simulink model "CryoDet12Chan"  (R2016b)
settings: Solver=ode45  StartTime=0.0  StopTime=10e-4  MaxStep=1e-9  RelTol=1e-3
values from neighbouring files (symbols this model uses):
  Fclk = Fadc/2    (= 153600000)    [setupCryoFPGA.m]    (also in setupCryoNew.m)
  freqBusAddrBits = 4    [setupCryoFPGA.m]    (also in setupCryoNew.m)
  noise = exp(2i*pi*rand(1, noiseLen))    [setupCryoFPGA.m]    (also in setupCryoNew.m)
  noiseLen = 128    [setupCryoFPGA.m]    (also in setupCryoNew.m)
  noiseSteps = 32    [setupCryoFPGA.m]    (also in setupCryoNew.m)
  notch = tf( [1 a*wNotch/Q wNotch^2], [1 wNotch/Q wNotch^2])    [setupCryoFPGA.m]    (also in setupCryoNew.m)
  notch2 = tf( [1 a*wNotch/Q wNotch^2], [1 wNotch/Q wNotch^2])    [setupCryoFPGA.m]    (also in setupCryoNew.m)
  notch3 = tf( [1 a*wNotch/Q wNotch^2], [1 wNotch/Q wNotch^2])    [setupCryoFPGA.m]    (also in setupCryoNew.m)
  notch4 = tf( [1 a*wNotch/Q wNotch^2], [1 wNotch/Q wNotch^2])    [setupCryoFPGA.m]    (also in setupCryoNew.m)
  Tclk = 1/Fclk    (= 6.51041666667e-09)    [setupCryoFPGA.m]    (also in setupCryoNew.m)
undefined symbols (not defined in the file or in its folder): AXI4, Lite, xlipgetpartsetting
libraries: xbsIndex_r4 x1191
(part 4 of 9)

== system CryoDet12Chan/DspCore/AdcDac 0/eta/Complex Divide ==
  note: Complex multiplier has latency 6
  a_tvalid : Inport
  A_Q : Inport  Port=2
  A_I : Inport  Port=3
  b_tvalid : Inport  Port=4
  B_Q : Inport  Port=5
  B_I : Inport  Port=6
  AddSub : xbsIndex_r4/AddSub  mode=Addition  use_carryin=off  use_carryout=off  en=off  latency=3  precision=Full  arith_type="Signed  (2's comp)"  n_bits=48  bin_pt=44  quantization=Truncate  overflow=Flag as error  use_behavioral_HDL=on  hw_selection=Fabric  pipelined=off  dbl_ovrd=off  block_type=addsub
  CMult : xbsIndex_r4/CMult  const=-1  gui_display_data_type=Floating-point  const_n_bits=16  const_bin_pt=15  float_type=Single  exp_bits=8  fraction_bits=24  en=off  latency=3  precision=Full  arith_type="Signed  (2's comp)"  n_bits=32  bin_pt=30  quantization=Truncate  overflow=Wrap  use_behavioral_HDL=off  mem_type=Distributed RAM  pipeline=off  dbl_ovrd=off  block_type=cmult
  Constant : xbsIndex_r4/Constant  const=0  gui_display_data_type=Floating-point  arith_type=Floating-point  n_bits=63  bin_pt=15  preci_type=Single  exp_width=8  frac_width=24  explicit_period=off  period=1  equ=P=C  opselect=C  inp2=PCIN>>17  opr=+  inp1=P  carry=CIN  dbl_ovrd=off  block_type=constant
  Cplx Div 2 : Scope  NumInputPorts=3
  CplxProd : Subsystem
  Cpx Div : Scope  NumInputPorts=4
  Delay{,1..2,5} (4 alike) : xbsIndex_r4/Delay  rst=off  infoeditControl=Selection of Reset will increase slice count due to use of real FFs and instead of SRLs  en=off  latency=3  reg_retiming=on  dbl_ovrd=off  block_type=delay
  Delay3 : xbsIndex_r4/Delay  rst=off  infoeditControl=Selection of Reset will increase slice count due to use of real FFs and instead of SRLs  en=off  latency=8  reg_retiming=on  dbl_ovrd=off  block_type=delay
  Divide : xbsIndex_r4/Divide  flow_control=NonBlocking  axi_optimize_goal=Resources  algorithm_type=Radix2  infoedit1=Specify output fraction-width for Fixed-point division.  fractional_width=24  infoedit2=Specify latency for Floating-point division.  latency=8  rate=1  has_a_tlast=off  has_a_tuser=off  has_b_tlast=off  has_b_tuser=off  en=off  has_result_tready=off  result_tlast_behv=Pass_A_TLAST  has_underflow=on  has_overflow=on  has_invalid_op=on  has_divide_by_zero=on  fpo_op_type=mergeddivide  block_type=divide
      settings: infoedit=Blocking: Wait for data on all inputs, allow back-pressure.<br>NonBlocking: operate every cycle in which all inputs are valid, no back-pressure.
  Divide1 : xbsIndex_r4/Divide  flow_control=NonBlocking  axi_optimize_goal=Resources  algorithm_type=Radix2  infoedit1=Specify output fraction-width for Fixed-point division.  fractional_width=24  infoedit2=Specify latency for Floating-point division.  latency=8  rate=1  has_a_tlast=off  has_a_tuser=off  has_b_tlast=off  has_b_tuser=off  en=off  has_result_tready=off  result_tlast_behv=Pass_A_TLAST  has_underflow=on  has_overflow=on  has_invalid_op=on  has_divide_by_zero=on  fpo_op_type=mergeddivide  block_type=divide
      settings: infoedit=Blocking: Wait for data on all inputs, allow back-pressure.<br>NonBlocking: operate every cycle in which all inputs are valid, no back-pressure.
  Gateway Out{6..17} (12 alike) : xbsIndex_r4/Gateway Out  inherit_from_input=off  hdl_port=off  rows=1  columns=1  UseAsDAC=off  DACChannel='1'  interface=None  automatic_assignment=on  address_offset=hex2dec('00')  intf_name=''  intf_description=''  timing_constraint=None  locs_specified=off  LOCs={}  io_standard={}  block_type=gatewayout
  Mult : xbsIndex_r4/Mult  precision=Full  arith_type="Signed  (2's comp)"  n_bits=48  bin_pt=44  quantization=Truncate  overflow=Flag as error  en=off  latency=6  use_behavioral_HDL=on  opt=Speed  use_embedded=on  optimum_pipeline=on  pipeline=on  dbl_ovrd=off  use_rpm=on  placement_style=Triangular  block_type=mult
  Mult1 : xbsIndex_r4/Mult  precision=Full  arith_type="Signed  (2's comp)"  n_bits=48  bin_pt=44  quantization=Truncate  overflow=Flag as error  en=off  latency=6  use_behavioral_HDL=on  opt=Speed  use_embedded=on  optimum_pipeline=off  pipeline=on  dbl_ovrd=off  use_rpm=on  placement_style=Triangular  block_type=mult
  Mux{1,3..5,8..10} (7 alike) : Mux  Inputs=2
  Mux6 : xbsIndex_r4/Mux  inputs=2  en=off  latency=0  precision=Full  arith_type=Unsigned  n_bits=63  bin_pt=15  quantization=Truncate  overflow=Flag as error  dbl_ovrd=off  block_type=mux
  Mux7 : xbsIndex_r4/Mux  inputs=2  en=off  latency=0  precision=Full  arith_type=Unsigned  n_bits=63  bin_pt=15  quantization=Truncate  overflow=Flag as error  dbl_ovrd=off  block_type=mux
  Terminator5 : Terminator
  tvalidOut : Outport
  Out_Q : Outport  Port=2
  Out_I : Outport  Port=3
  invalid op : Outport  Port=4
  wires:
  a_tvalid/1 -> Gateway Out13/1, Gateway Out12/1, Delay/1
  A_Q/1 -> Delay1/1, Gateway Out14/1
  A_I/1 -> Delay2/1, Gateway Out15/1
  Divide/1 -> Mux7/2
  Mult1/1 -> AddSub/2
  AddSub/1 -> Divide/2, Divide1/2
  Divide1/4 -> Gateway Out11/1, invalid op/1, Mux6/1, Mux7/1
  Mux7/1 -> Gateway Out6/1, Out_Q/1
  Mux6/1 -> Out_I/1, Gateway Out7/1
  Mult/1 -> AddSub/1
  Gateway Out6/1 -> Mux3/1
  Gateway Out7/1 -> Mux3/2
  Gateway Out8/1 -> Mux4/1
  Gateway Out9/1 -> Mux4/2
  Gateway Out10/1 -> Mux5/1
  Gateway Out11/1 -> Mux5/2
  Divide1/1 -> Mux6/2
  Constant/1 -> Mux7/3, Mux6/3
  Delay5/1 -> CplxProd/5(Re_B)
  Delay2/1 -> CplxProd/3(Re_A)
  Delay1/1 -> CplxProd/2(Im_A)
  Delay/1 -> CplxProd/1(tvalidIn)
  B_Q/1 -> Mult1/1, Mult1/2, Gateway Out16/1, CMult/1
  B_I/1 -> Mult/1, Mult/2, Delay5/1, Gateway Out17/1
  CMult/1 -> CplxProd/4(Im_B)
  Gateway Out12/1 -> Mux8/1
  Gateway Out13/1 -> Mux8/2
  Gateway Out14/1 -> Mux9/1
  Gateway Out15/1 -> Mux9/2
  Gateway Out16/1 -> Mux10/1
  Gateway Out17/1 -> Mux10/2
  Mux8/1 -> Cplx Div 2/1
  Mux9/1 -> Cplx Div 2/2
  Mux10/1 -> Cplx Div 2/3
  b_tvalid/1 -> Terminator5/1
  CplxProd/2(Im_Out) -> Divide/1
  CplxProd/1(tvalidOut) -> Mux1/2, Delay3/1
  CplxProd/3(Re_Out) -> Divide1/1
  Divide1/2 -> Gateway Out8/1
  Divide1/3 -> Gateway Out9/1
  Divide1/5 -> Gateway Out10/1
  Mux3/1 -> Cpx Div/2
  Mux4/1 -> Cpx Div/3
  Mux5/1 -> Cpx Div/4
  Delay3/1 -> Mux1/1, tvalidOut/1
  Mux1/1 -> Cpx Div/1

== system CryoDet12Chan/DspCore/AdcDac 0/eta/CplxProd ==
  tvalidIn : Inport
  Im_A : Inport  Port=2
  Re_A : Inport  Port=3
  Im_B : Inport  Port=4
  Re_B : Inport  Port=5
  AddSub : xbsIndex_r4/AddSub  mode=Subtraction  use_carryin=off  use_carryout=off  en=off  latency=3  precision=Full  arith_type=Unsigned  n_bits=16  bin_pt=14  quantization=Truncate  overflow=Wrap  use_behavioral_HDL=off  hw_selection=DSP48  pipelined=on  dbl_ovrd=off  block_type=addsub
  AddSub1 : xbsIndex_r4/AddSub  mode=Addition  use_carryin=off  use_carryout=off  en=off  latency=3  precision=Full  arith_type=Unsigned  n_bits=16  bin_pt=14  quantization=Truncate  overflow=Wrap  use_behavioral_HDL=off  hw_selection=DSP48  pipelined=on  dbl_ovrd=off  block_type=addsub
  Delay : xbsIndex_r4/Delay  rst=off  infoeditControl=Selection of Reset will increase slice count due to use of real FFs and instead of SRLs  en=off  latency=3  reg_retiming=off  dbl_ovrd=off  block_type=delay
  Delay1 : xbsIndex_r4/Delay  rst=off  infoeditControl=Selection of Reset will increase slice count due to use of real FFs and instead of SRLs  en=off  latency=3  reg_retiming=off  dbl_ovrd=off  block_type=delay
  Mult{,1..3} (4 alike) : xbsIndex_r4/Mult  precision=Full  arith_type="Signed  (2's comp)"  n_bits=16  bin_pt=14  quantization=Truncate  overflow=Wrap  en=off  latency=3  use_behavioral_HDL=off  opt=Speed  use_embedded=on  optimum_pipeline=off  pipeline=on  dbl_ovrd=off  use_rpm=on  placement_style=Triangular  block_type=mult
  tvalidOut : Outport
  Im_Out : Outport  Port=2
  Re_Out : Outport  Port=3
  wires:
  Delay/1 -> Delay1/1
  Mult2/1 -> AddSub1/1
  Mult/1 -> AddSub/1
  Mult1/1 -> AddSub/2
  Mult3/1 -> AddSub1/2
  Re_A/1 -> Mult3/1, Mult/1
  Im_A/1 -> Mult2/1, Mult1/1
  tvalidIn/1 -> Delay/1
  Im_B/1 -> Mult1/2, Mult3/2
  Re_B/1 -> Mult/2, Mult2/2
  Delay1/1 -> tvalidOut/1
  AddSub/1 -> Re_Out/1
  AddSub1/1 -> Im_Out/1

== system CryoDet12Chan/DspCore/AdcDac 0/eta/CplxProd1 ==
  tvalidIn : Inport
  Im_A : Inport  Port=2
  Re_A : Inport  Port=3
  Im_B : Inport  Port=4
  Re_B : Inport  Port=5
  AddSub : xbsIndex_r4/AddSub  mode=Subtraction  use_carryin=off  use_carryout=off  en=off  latency=3  precision=Full  arith_type=Unsigned  n_bits=16  bin_pt=14  quantization=Truncate  overflow=Wrap  use_behavioral_HDL=off  hw_selection=DSP48  pipelined=on  dbl_ovrd=off  block_type=addsub
  AddSub1 : xbsIndex_r4/AddSub  mode=Addition  use_carryin=off  use_carryout=off  en=off  latency=3  precision=Full  arith_type=Unsigned  n_bits=16  bin_pt=14  quantization=Truncate  overflow=Wrap  use_behavioral_HDL=off  hw_selection=DSP48  pipelined=on  dbl_ovrd=off  block_type=addsub
  Delay : xbsIndex_r4/Delay  rst=off  infoeditControl=Selection of Reset will increase slice count due to use of real FFs and instead of SRLs  en=off  latency=3  reg_retiming=off  dbl_ovrd=off  block_type=delay
  Delay1 : xbsIndex_r4/Delay  rst=off  infoeditControl=Selection of Reset will increase slice count due to use of real FFs and instead of SRLs  en=off  latency=3  reg_retiming=off  dbl_ovrd=off  block_type=delay
  Mult{,1..3} (4 alike) : xbsIndex_r4/Mult  precision=Full  arith_type="Signed  (2's comp)"  n_bits=16  bin_pt=14  quantization=Truncate  overflow=Wrap  en=off  latency=3  use_behavioral_HDL=off  opt=Speed  use_embedded=on  optimum_pipeline=off  pipeline=on  dbl_ovrd=off  use_rpm=on  placement_style=Triangular  block_type=mult
  tvalidOut : Outport
  Im_Out : Outport  Port=2
  Re_Out : Outport  Port=3
  wires:
  Delay/1 -> Delay1/1
  Mult2/1 -> AddSub1/1
  Mult/1 -> AddSub/1
  Mult1/1 -> AddSub/2
  Mult3/1 -> AddSub1/2
  Re_A/1 -> Mult3/1, Mult/1
  Im_A/1 -> Mult2/1, Mult1/1
  tvalidIn/1 -> Delay/1
  Im_B/1 -> Mult1/2, Mult3/2
  Re_B/1 -> Mult/2, Mult2/2
  Delay1/1 -> tvalidOut/1
  AddSub/1 -> Re_Out/1
  AddSub1/1 -> Im_Out/1

== system CryoDet12Chan/DspCore/AdcDac 0/eta/CplxProd2 ==
  tvalidIn : Inport
  Im_A : Inport  Port=2
  Re_A : Inport  Port=3
  Im_B : Inport  Port=4
  Re_B : Inport  Port=5
  AddSub : xbsIndex_r4/AddSub  mode=Subtraction  use_carryin=off  use_carryout=off  en=off  latency=3  precision=Full  arith_type=Unsigned  n_bits=16  bin_pt=14  quantization=Truncate  overflow=Wrap  use_behavioral_HDL=off  hw_selection=DSP48  pipelined=on  dbl_ovrd=off  block_type=addsub
  AddSub1 : xbsIndex_r4/AddSub  mode=Addition  use_carryin=off  use_carryout=off  en=off  latency=3  precision=Full  arith_type=Unsigned  n_bits=16  bin_pt=14  quantization=Truncate  overflow=Wrap  use_behavioral_HDL=off  hw_selection=DSP48  pipelined=on  dbl_ovrd=off  block_type=addsub
  Delay : xbsIndex_r4/Delay  rst=off  infoeditControl=Selection of Reset will increase slice count due to use of real FFs and instead of SRLs  en=off  latency=3  reg_retiming=off  dbl_ovrd=off  block_type=delay
  Delay1 : xbsIndex_r4/Delay  rst=off  infoeditControl=Selection of Reset will increase slice count due to use of real FFs and instead of SRLs  en=off  latency=3  reg_retiming=off  dbl_ovrd=off  block_type=delay
  Mult{,1..3} (4 alike) : xbsIndex_r4/Mult  precision=Full  arith_type="Signed  (2's comp)"  n_bits=16  bin_pt=14  quantization=Truncate  overflow=Wrap  en=off  latency=3  use_behavioral_HDL=off  opt=Speed  use_embedded=on  optimum_pipeline=off  pipeline=on  dbl_ovrd=off  use_rpm=on  placement_style=Triangular  block_type=mult
  tvalidOut : Outport
  Im_Out : Outport  Port=2
  Re_Out : Outport  Port=3
  wires:
  Delay/1 -> Delay1/1
  Mult2/1 -> AddSub1/1
  Mult/1 -> AddSub/1
  Mult1/1 -> AddSub/2
  Mult3/1 -> AddSub1/2
  Re_A/1 -> Mult3/1, Mult/1
  Im_A/1 -> Mult2/1, Mult1/1
  tvalidIn/1 -> Delay/1
  Im_B/1 -> Mult1/2, Mult3/2
  Re_B/1 -> Mult/2, Mult2/2
  Delay1/1 -> tvalidOut/1
  AddSub/1 -> Re_Out/1
  AddSub1/1 -> Im_Out/1

== system CryoDet12Chan/DspCore/AdcDac 0/eta/LPF ==
  note: REF channel should not be low-passed!
      | Needs to have same bandwidth as signal channel
      | but latency must match
  note: streaming interface? so complex divide gets data at lower rate?
  note: tvalid
  note: Channel #
  note: Sig+
  note: Sig-
  note: Ref+
  note: Ref
  note: Sig
  note: Ref-
  In1 : Inport
  Bus Creator : BusCreator  Inputs=2
  Bus Creator1 : BusCreator  Inputs=2
  Bus Selector : BusSelector  OutputSignals=chanAndTvalid,signal2
  Bus Selector1 : BusSelector  OutputSignals=channel,valid
  Bus Selector2 : BusSelector  OutputSignals=channel,tvalid
  CIC Compiler 4.0 {1..10} (10 alike) : xbsIndex_r4/CIC Compiler 4.0   filter_type=Decimation  number_of_stages=3  differential_delay=1  number_of_channels=12  sample_rate_changes=Fixed  fixed_or_initial_rate=8  minimum_rate=8  maximum_rate=8  ratespecification=Sample_Period  sampleperiod=1  hardwareoversamplingrate=1  quantization=Truncation  output_data_width=24  use_xtreme_dsp_slice=off  use_streaming_interface=on  has_aclken=off  has_aresetn=on  has_dout_tready=off  trim_axipin_name=on  gui_behaviour=Sysgen_GUI  input_data_width=18  ip_name=CIC Compiler  ip_version=4.0  dsptool_ready=true  wrapper_available=true  port_translation_map={ 'aclken' => 'en', 'aresetn' => 'rst' }  ipcore_xco_need_fpga_part=true  ipcore_verbose=false  block_type=cic_compiler_v4_0
  CIC LPF Scope : Scope  NumInputPorts=6
  CIC LPF input scope : Scope  NumInputPorts=5
  CIC reset : Subsystem
  Constant4 : xbsIndex_r4/Constant  const=10  gui_display_data_type=Fixed-point  arith_type=Unsigned  n_bits=4  bin_pt=0  preci_type=Single  exp_width=8  frac_width=24  explicit_period=off  period=1  equ=P=C  opselect=C  inp2=PCIN>>17  opr=+  inp1=P  carry=CIN  dbl_ovrd=off  block_type=constant
  Demux{,3..6} (5 alike) : Demux  Outputs=2
  Demux1 : Demux  Outputs=6
  Display : Display
  Gateway Out{,1,5..18} (16 alike) : xbsIndex_r4/Gateway Out  inherit_from_input=off  hdl_port=off  rows=1  columns=1  UseAsDAC=off  DACChannel='1'  interface=None  automatic_assignment=on  address_offset=hex2dec('00')  intf_name=''  intf_description=''  timing_constraint=None  locs_specified=off  LOCs={}  io_standard={}  block_type=gatewayout
  LPF chan output : Scope  NumInputPorts=2
  Mux : Mux  Inputs=2
  Mux1 : Mux  Inputs=10
  Mux3 : Mux  Inputs=2
  Mux4 : Mux  Inputs=2
  Scale{,1..9} (10 alike) : xbsIndex_r4/Scale  scale_factor=-9  dbl_ovrd=off  block_type=scale
  Terminator : Terminator
  Out1 : Outport
  wires:
  Demux1/1 -> Terminator/1
  Demux1/2 -> Demux/1
  Demux1/3 -> Demux3/1
  Demux1/5 -> Demux5/1
  Demux1/6 -> Demux6/1
  Bus Selector/2 -> Demux1/1  "<signal2>"
  In1/1 -> Bus Selector/1
  Demux1/4 -> Demux4/1
  Demux/1 -> Gateway Out16/1, CIC Compiler 4.0 3/2
  Demux/2 -> CIC Compiler 4.0 1/2
  Demux3/1 -> CIC Compiler 4.0 2/2
  Demux3/2 -> CIC Compiler 4.0 4/2
  Demux5/1 -> CIC Compiler 4.0 7/2
  Demux5/2 -> CIC Compiler 4.0 8/2
  Demux6/1 -> CIC Compiler 4.0 9/2
  Demux6/2 -> CIC Compiler 4.0 10/2
  Bus Selector1/2 -> CIC Compiler 4.0 3/1, CIC Compiler 4.0 1/1, CIC Compiler 4.0 2/1, CIC Compiler 4.0 4/1, CIC Compiler 4.0 5/1, CIC Compiler 4.0 6/1, CIC Compiler 4.0 7/1, CIC Compiler 4.0 8/1, CIC Compiler 4.0 9/1, CIC Compiler 4.0 10/1  "<valid>"
  Bus Selector1/1 -> Gateway Out15/1, CIC reset/2(Channel), [ChanIn]  "<channel>"
  Bus Selector/1 -> Bus Selector1/1  "<chanAndTvalid>"
  CIC Compiler 4.0 3/3 -> Scale/1
  CIC Compiler 4.0 1/3 -> Scale1/1
  CIC Compiler 4.0 2/3 -> Scale2/1
  CIC Compiler 4.0 4/3 -> Scale3/1
  Demux4/1 -> CIC Compiler 4.0 5/2
  Demux4/2 -> CIC Compiler 4.0 6/2
  CIC Compiler 4.0 7/3 -> Scale4/1
  CIC Compiler 4.0 8/3 -> Scale5/1
  CIC Compiler 4.0 9/3 -> Scale6/1
  CIC Compiler 4.0 10/3 -> Scale7/1
  Mux1/1 -> Bus Creator/2
  Bus Creator/1 -> Out1/1
  Bus Creator1/1 -> Bus Creator/1, Bus Selector2/1
  Scale/1 -> Gateway Out1/1, Mux1/1
  Scale1/1 -> Mux1/2
  Scale2/1 -> Mux1/3
  Scale3/1 -> Mux1/4
  Scale4/1 -> Mux1/7
  Scale5/1 -> Mux1/8
  Scale6/1 -> Mux1/9
  Scale7/1 -> Mux1/10
  CIC Compiler 4.0 7/2 -> Bus Creator1/2  "tvalid"
  Scale8/1 -> Mux1/5
  Scale9/1 -> Mux1/6
  CIC Compiler 4.0 4/6 -> Gateway Out/1
  CIC Compiler 4.0 7/6 -> Bus Creator1/1  "channel"
  CIC Compiler 4.0 3/1 -> Gateway Out5/1
  CIC Compiler 4.0 3/2 -> Gateway Out6/1
  CIC Compiler 4.0 3/4 -> Gateway Out7/1
  CIC Compiler 4.0 3/5 -> Gateway Out8/1
  CIC Compiler 4.0 3/6 -> Gateway Out9/1
  CIC Compiler 4.0 3/7 -> Gateway Out10/1
  CIC Compiler 4.0 3/8 -> Gateway Out11/1
  Gateway Out11/1 -> Mux3/2
  Gateway Out10/1 -> Mux3/1
  Mux3/1 -> CIC LPF Scope/6
  Gateway Out9/1 -> CIC LPF Scope/5
  Gateway Out8/1 -> CIC LPF Scope/4
  Gateway Out7/1 -> CIC LPF Scope/3
  Gateway Out6/1 -> CIC LPF Scope/2
  CIC reset/1(notResetOut) -> Gateway Out18/1, CIC Compiler 4.0 3/4, CIC Compiler 4.0 1/4, CIC Compiler 4.0 2/4, CIC Compiler 4.0 4/4, CIC Compiler 4.0 5/4, CIC Compiler 4.0 6/4, CIC Compiler 4.0 7/4, CIC Compiler 4.0 8/4, CIC Compiler 4.0 9/4, CIC Compiler 4.0 10/4
  Constant4/1 -> CIC reset/3(N-2)
  [fpgaReset] -> Gateway Out14/1, CIC reset/1(resetIn)
  CIC reset/2(tlast) -> CIC Compiler 4.0 2/3, CIC Compiler 4.0 5/3, CIC Compiler 4.0 6/3, CIC Compiler 4.0 8/3, CIC Compiler 4.0 9/3, CIC Compiler 4.0 10/3, CIC Compiler 4.0 7/3, CIC Compiler 4.0 4/3, CIC Compiler 4.0 3/3, Gateway Out17/1, CIC Compiler 4.0 1/3
  Gateway Out18/1 -> CIC LPF input scope/5
  Gateway Out17/1 -> CIC LPF input scope/4
  Gateway Out16/1 -> CIC LPF input scope/3
  Gateway Out15/1 -> CIC LPF input scope/2
  Gateway Out14/1 -> CIC LPF input scope/1
  Gateway Out5/1 -> Mux4/2
  Gateway Out1/1 -> Mux4/1
  Mux4/1 -> CIC LPF Scope/1
  Bus Selector2/2 -> Gateway Out13/1  "<tvalid>"
  Bus Selector2/1 -> Gateway Out12/1  "<channel>"
  Gateway Out12/1 -> Mux/1
  Gateway Out13/1 -> Mux/2
  Mux/1 -> LPF chan output/1
  Gateway Out/1 -> LPF chan output/2, Display/1
  CIC Compiler 4.0 5/3 -> Scale8/1
  CIC Compiler 4.0 6/3 -> Scale9/1

== system CryoDet12Chan/DspCore/AdcDac 0/loopFilter/initial Frequencies ==
  note: Channel 15 used for none of above
  note: initial Frequencies
  note: select initial frequency
      | for now just mux from input registers
      | eventually configure RAM and loading protocol
  channel : Inport
  Gateway Out12 : xbsIndex_r4/Gateway Out  inherit_from_input=off  hdl_port=off  rows=1  columns=1  UseAsDAC=off  DACChannel='1'  interface=None  automatic_assignment=on  address_offset=hex2dec('00')  intf_name=''  intf_description=''  timing_constraint=None  locs_specified=off  LOCs={}  io_standard={}  block_type=gatewayout
  Gateway Out13 : xbsIndex_r4/Gateway Out  inherit_from_input=off  hdl_port=off  rows=1  columns=1  UseAsDAC=off  DACChannel='1'  interface=None  automatic_assignment=on  address_offset=hex2dec('00')  intf_name=''  intf_description=''  timing_constraint=None  locs_specified=off  LOCs={}  io_standard={}  block_type=gatewayout
  Mux : xbsIndex_r4/Mux  inputs=16  en=off  latency=0  precision=Full  arith_type=Unsigned  n_bits=24  bin_pt=24  quantization=Truncate  overflow=Wrap  dbl_ovrd=off  block_type=mux
  initial Freqs : Scope  NumInputPorts=2
  Fi : Outport
  wires:
  channel/1 -> Gateway Out12/1, Mux/1
  [F0] -> Mux/2
  [F1] -> Mux/3
  [F2] -> Mux/4
  [F3] -> Mux/5
  [F4] -> Mux/6
  [F5] -> Mux/7
  [F6] -> Mux/8
  [F7] -> Mux/9
  [F8] -> Mux/10
  [F9] -> Mux/11
  [F10] -> Mux/12
  [F11] -> Mux/14, Mux/15, Mux/16, Mux/17, Mux/13
  Mux/1 -> Gateway Out13/1, Fi/1
  Gateway Out13/1 -> initial Freqs/2
  Gateway Out12/1 -> initial Freqs/1

== system CryoDet12Chan/DspCore/AdcDac 0/twelveLineUDC 0/DAC Sum ==
  note: Final adder stages reduce to 16 bits
  note: DAC1 (odd samples)
  note: DAC0 (even samples)
  In1 : Inport
  In2 : Inport  Port=2
  In3 : Inport  Port=3
  In4 : Inport  Port=4
  In5 : Inport  Port=5
  In6 : Inport  Port=6
  In7 : Inport  Port=7
  In8 : Inport  Port=8
  In9 : Inport  Port=9
  In10 : Inport  Port=10
  In11 : Inport  Port=11
  In12 : Inport  Port=12
  AddSub{,1..19} (20 alike) : xbsIndex_r4/AddSub  mode=Addition  use_carryin=off  use_carryout=off  en=off  latency=3  precision=User Defined  arith_type="Signed  (2's comp)"  n_bits=20  bin_pt=15  quantization=Truncate  overflow=Wrap  use_behavioral_HDL=off  hw_selection=Fabric  pipelined=off  dbl_ovrd=off  block_type=addsub
  AddSub20 : xbsIndex_r4/AddSub  mode=Addition  use_carryin=off  use_carryout=off  en=off  latency=3  precision=User Defined  arith_type="Signed  (2's comp)"  n_bits=16  bin_pt=15  quantization="Round  (unbiased: +/- Inf)"  overflow=Saturate  use_behavioral_HDL=off  hw_selection=Fabric  pipelined=off  dbl_ovrd=off  block_type=addsub
  AddSub21 : xbsIndex_r4/AddSub  mode=Addition  use_carryin=off  use_carryout=off  en=off  latency=3  precision=User Defined  arith_type="Signed  (2's comp)"  n_bits=16  bin_pt=15  quantization="Round  (unbiased: +/- Inf)"  overflow=Saturate  use_behavioral_HDL=off  hw_selection=Fabric  pipelined=off  dbl_ovrd=off  block_type=addsub
  DAC sum scope : Scope  NumInputPorts=2
  DAC sum scope1 : Scope  NumInputPorts=6
  Demux{,1..11} (12 alike) : Demux  Outputs=2
  Gateway Out{,1..9} (10 alike) : xbsIndex_r4/Gateway Out  inherit_from_input=off  hdl_port=off  rows=1  columns=1  UseAsDAC=off  DACChannel='1'  interface=None  automatic_assignment=on  address_offset=hex2dec('00')  intf_name=''  intf_description=''  timing_constraint=None  locs_specified=off  LOCs={}  io_standard={}  block_type=gatewayout
  Mux : Mux  Inputs=2
  Mux1 : Mux  Inputs=2
  Mux2 : Mux  Inputs=2
  Out1 : Outport
  wires:
  In1/1 -> Demux1/1
  In2/1 -> Demux/1
  In3/1 -> Demux2/1
  In4/1 -> Demux3/1
  In5/1 -> Demux4/1
  In6/1 -> Demux5/1
  In7/1 -> Demux6/1
  In8/1 -> Demux7/1
  In9/1 -> Demux8/1
  In10/1 -> Demux9/1
  In11/1 -> Demux10/1
  Demux/1 -> Gateway Out5/1, AddSub/2
  Demux2/1 -> Gateway Out6/1, AddSub2/1
  Demux3/1 -> Gateway Out7/1, AddSub2/2
  Demux4/1 -> Gateway Out8/1, AddSub4/1
  Demux5/1 -> Gateway Out9/1, AddSub4/2
  Demux6/1 -> AddSub6/1
  Demux8/1 -> AddSub8/1
  In12/1 -> Demux11/1
  AddSub20/1 -> Mux/1
  AddSub21/1 -> Mux/2
  Mux/1 -> Out1/1
  Demux7/1 -> AddSub6/2
  Demux9/1 -> AddSub8/2
  Demux10/1 -> AddSub10/1
  Demux11/1 -> AddSub10/2
  Demux/2 -> AddSub1/1
  Demux1/2 -> AddSub1/2
  Demux11/2 -> AddSub11/1
  Demux10/2 -> AddSub11/2
  Demux9/2 -> AddSub9/1
  Demux8/2 -> AddSub9/2
  Demux7/2 -> AddSub7/1
  Demux6/2 -> AddSub7/2
  Demux5/2 -> AddSub5/1
  Demux4/2 -> AddSub5/2
  Demux3/2 -> AddSub3/1
  Demux2/2 -> AddSub3/2
  AddSub/1 -> AddSub12/1
  AddSub2/1 -> AddSub12/2
  AddSub4/1 -> AddSub13/1
  AddSub6/1 -> AddSub13/2
  AddSub8/1 -> AddSub14/1
  AddSub10/1 -> AddSub14/2
  AddSub12/1 -> AddSub15/1
  AddSub13/1 -> AddSub15/2
  AddSub15/1 -> AddSub20/1, Gateway Out/1
  AddSub14/1 -> Gateway Out1/1, AddSub20/2
  AddSub1/1 -> AddSub16/1
  AddSub3/1 -> AddSub16/2
  AddSub5/1 -> AddSub17/1
  AddSub7/1 -> AddSub17/2
  AddSub9/1 -> AddSub18/1
  AddSub11/1 -> AddSub18/2
  AddSub16/1 -> AddSub19/1
  AddSub17/1 -> AddSub19/2
  AddSub19/1 -> Gateway Out2/1, AddSub21/1
  AddSub18/1 -> AddSub21/2, Gateway Out3/1
  Gateway Out3/1 -> Mux2/2
  Gateway Out2/1 -> Mux2/1
  Gateway Out1/1 -> Mux1/2
  Gateway Out/1 -> Mux1/1
  Mux1/1 -> DAC sum scope/1
  Mux2/1 -> DAC sum scope/2
  Gateway Out4/1 -> DAC sum scope1/1
  Gateway Out5/1 -> DAC sum scope1/2
  Gateway Out6/1 -> DAC sum scope1/3
  Gateway Out7/1 -> DAC sum scope1/4
  Gateway Out8/1 -> DAC sum scope1/5
  Gateway Out9/1 -> DAC sum scope1/6
  Demux1/1 -> Gateway Out4/1, AddSub/1

== system CryoDet12Chan/DspCore/AdcDac 0/twelveLineUDC 0/Mux12X4 ==
  note: I think this will select a channel 1 or 2 ticks after it has updated,
      | which should work fine. But optimal would be to delay synch in by 11 ticks = N-1
  note: Channel ID
  note: Reference Q&I
  note: Signal Q&I
  note: Twelve busses 4-wide each time-division multiplexed onto a 4-wide bus
  line0 : Inport
  line1 : Inport  Port=2
  line2 : Inport  Port=3
  line3 : Inport  Port=4
  line4 : Inport  Port=5
  line5 : Inport  Port=6
  line6 : Inport  Port=7
  line7 : Inport  Port=8
  line8 : Inport  Port=9
  line9 : Inport  Port=10
  line10 : Inport  Port=11
  line11 : Inport  Port=12
  synch : Inport  Port=13
  "12x4 Mux out scope " : Scope  NumInputPorts=3
  Bus Creator : BusCreator  Inputs=2
  Counter : xbsIndex_r4/Counter  cnt_type=Count Limited  cnt_to=11  operation=Up  start_count=0  cnt_by_val=1  arith_type=Unsigned  n_bits=4  bin_pt=0  load_pin=off  rst=on  en=off  explicit_period=off  period=Tclk  use_behavioral_HDL=off  implementation=Fabric  dbl_ovrd=off  block_type=counter
  Delay1 : xbsIndex_r4/Delay  rst=off  infoeditControl=Selection of Reset will increase slice count due to use of real FFs and instead of SRLs  en=off  latency=1  reg_retiming=off  dbl_ovrd=off  block_type=delay
  Demux{,1..11} (12 alike) : Demux
  Gateway Out{1..8} (8 alike) : xbsIndex_r4/Gateway Out  inherit_from_input=off  hdl_port=off  rows=1  columns=1  UseAsDAC=off  DACChannel='1'  interface=None  automatic_assignment=on  address_offset=hex2dec('00')  intf_name=''  intf_description=''  timing_constraint=None  locs_specified=off  LOCs={}  io_standard={}  block_type=gatewayout
  Mux{,1..3} (4 alike) : xbsIndex_r4/Mux  inputs=12  en=off  latency=1  precision=Full  arith_type=Unsigned  n_bits=16  bin_pt=14  quantization=Truncate  overflow=Wrap  dbl_ovrd=off  block_type=mux
  Mux{4..9} (6 alike) : Mux  Inputs=2
  debug synch Scope : Scope  NumInputPorts=2
  Out1 : Outport
  wires:
  line0/1 -> Demux/1
  line5/1 -> Demux6/1
  line4/1 -> Demux5/1
  line3/1 -> Demux4/1
  line2/1 -> Demux3/1
  line1/1 -> Demux1/1
  Demux/1 -> Gateway Out4/1, Mux/2
  Demux/2 -> Mux1/2
  Demux/3 -> Mux2/2
  Demux/4 -> Mux3/2
  Demux1/1 -> Mux/3
  Demux1/2 -> Mux1/3
  Demux1/3 -> Mux2/3
  Demux1/4 -> Mux3/3
  Demux3/1 -> Mux/4
  Demux3/2 -> Mux1/4
  Demux3/3 -> Mux2/4
  Demux3/4 -> Mux3/4
  line11/1 -> Demux11/1
  line10/1 -> Demux10/1
  line9/1 -> Demux9/1
  line8/1 -> Demux8/1
  line7/1 -> Demux7/1
  line6/1 -> Demux2/1
  Demux4/1 -> Mux/5
  Demux4/2 -> Mux1/5
  Demux4/3 -> Mux2/5
  Demux4/4 -> Mux3/5
  Demux5/1 -> Mux/6
  Demux5/2 -> Mux1/6
  Demux5/3 -> Mux2/6
  Demux5/4 -> Mux3/6
  Demux6/1 -> Mux/7
  Demux6/2 -> Mux1/7
  Demux6/3 -> Mux2/7
  Demux6/4 -> Mux3/7
  Demux2/1 -> Mux/8
  Demux2/3 -> Mux2/8
  Demux2/4 -> Mux3/8
  Demux7/1 -> Mux/9
  Demux7/2 -> Mux1/9
  Demux2/2 -> Mux1/8
  Demux7/3 -> Mux2/9
  Demux7/4 -> Mux3/9
  Demux8/1 -> Mux/10
  Demux8/2 -> Mux1/10
  Demux8/3 -> Mux2/10
  Demux8/4 -> Mux3/10
  Demux9/1 -> Mux/11
  Demux9/2 -> Mux1/11
  Demux9/3 -> Mux2/11
  Demux9/4 -> Mux3/11
  Demux10/1 -> Mux/12
  Demux10/2 -> Mux1/12
  Demux10/3 -> Mux2/12
  Demux10/4 -> Mux3/12
  Demux11/1 -> Mux/13
  Demux11/2 -> Mux1/13
  Demux11/3 -> Mux2/13
  Demux11/4 -> Mux3/13
  synch/1 -> Gateway Out8/1, Counter/1
  Mux/1 -> Gateway Out2/1, Mux6/1
  Mux1/1 -> Gateway Out3/1, Mux6/2
  Mux2/1 -> Gateway Out6/1, Mux5/1
  Mux3/1 -> Gateway Out7/1, Mux5/2
  Mux6/1 -> Mux4/1
  Mux5/1 -> Mux4/2
  Counter/1 -> Mux2/1, Delay1/1, Mux1/1, Mux3/1, Mux/1, Gateway Out5/1
  Mux4/1 -> Bus Creator/2
  Delay1/1 -> Gateway Out1/1, Bus Creator/1  "channel"
  Bus Creator/1 -> Out1/1
  Gateway Out7/1 -> Mux7/2
  Gateway Out6/1 -> Mux7/1
  Gateway Out3/1 -> Mux8/2
  Gateway Out2/1 -> Mux8/1
  Mux7/1 -> "12x4 Mux out scope "/3
  Mux8/1 -> "12x4 Mux out scope "/2
  Gateway Out1/1 -> "12x4 Mux out scope "/1
  Gateway Out8/1 -> debug synch Scope/2
  Gateway Out4/1 -> Mux9/2
  Mux9/1 -> debug synch Scope/1
  Gateway Out5/1 -> Mux9/1

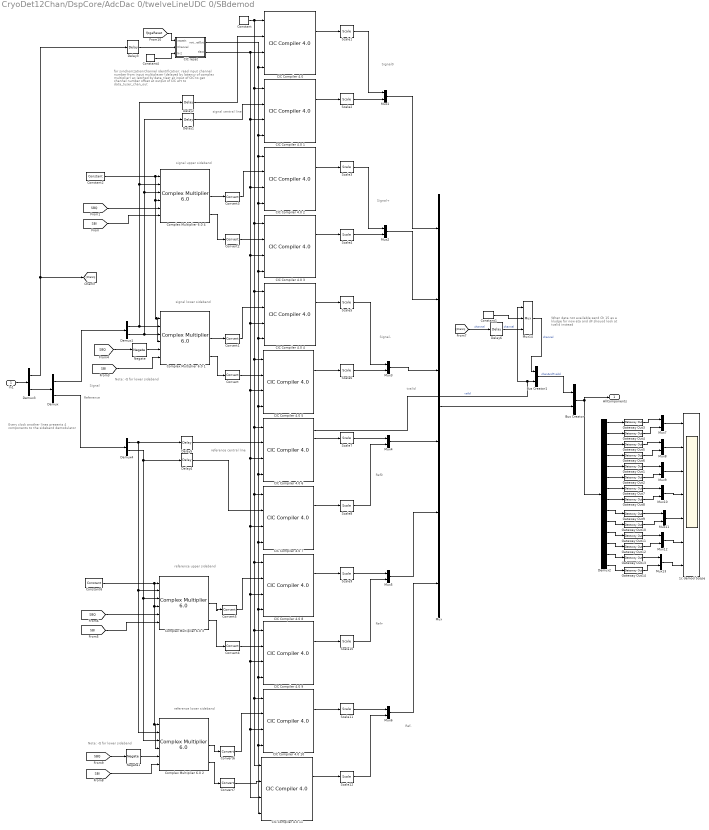
== system CryoDet12Chan/DspCore/AdcDac 0/twelveLineUDC 0/SBdemod ==
  note: When data not available send Ch 15 as
      | a kludge for now
      | eta and dF shouod look at tvalid instead
  note: tvalid
  note: Ref-
  note: Ref+
  note: Ref0
  note: Signal-
  note: Signal+
  note: Signal0
  note: for synchonization/channel identification:
      | read input channel number  from input multiplexer (delayed by latency of complex multiplier)
      | as latched by data_tlast at input of CIC to get channel number offset at output of CIC wrt to data_tuser_chan_out
  note: Note: -Q for lower sideband
  note: Every clock another lines presents 4 components to the sideband demodulator
  note: signal
      | central line
  note: signal
      | upper sideband
  note: signal
      | lower sideband
  note: Signal
  note: Reference
  note: reference
      | central line
  note: reference
      | upper sideband
  note: reference
      | lower sideband
  note: Note: -Q for lower sideband
  In1 : Inport
  1c demod Scope : Scope  NumInputPorts=7
  Bus Creator : BusCreator  Inputs=2
  Bus Creator1 : BusCreator  Inputs=2
  CIC Compiler 4.0 {,1..5,7..11} (11 alike) : xbsIndex_r4/CIC Compiler 4.0   filter_type=Decimation  number_of_stages=3  differential_delay=1  number_of_channels=12  sample_rate_changes=Fixed  fixed_or_initial_rate=12  minimum_rate=12  maximum_rate=12  ratespecification=Sample_Period  sampleperiod=1  hardwareoversamplingrate=1  quantization=Truncation  output_data_width=24  use_xtreme_dsp_slice=off  use_streaming_interface=off  has_aclken=off  has_aresetn=on  has_dout_tready=off  trim_axipin_name=on  gui_behaviour=Sysgen_GUI  input_data_width=18  ip_name=CIC Compiler  ip_version=4.0  dsptool_ready=true  wrapper_available=true  port_translation_map={ 'aclken' => 'en', 'aresetn' => 'rst' }  ipcore_xco_need_fpga_part=true  ipcore_verbose=false  block_type=cic_compiler_v4_0
  CIC Compiler 4.0 6 : xbsIndex_r4/CIC Compiler 4.0   filter_type=Decimation  number_of_stages=3  differential_delay=1  number_of_channels=12  sample_rate_changes=Fixed  fixed_or_initial_rate=12  minimum_rate=12  maximum_rate=12  ratespecification=Sample_Period  sampleperiod=1  hardwareoversamplingrate=2  quantization=Truncation  output_data_width=24  use_xtreme_dsp_slice=off  use_streaming_interface=off  has_aclken=off  has_aresetn=on  has_dout_tready=off  trim_axipin_name=on  gui_behaviour=Sysgen_GUI  input_data_width=18  ip_name=CIC Compiler  ip_version=4.0  dsptool_ready=true  wrapper_available=true  port_translation_map={ 'aclken' => 'en', 'aresetn' => 'rst' }  ipcore_xco_need_fpga_part=true  ipcore_verbose=false  block_type=cic_compiler_v4_0
  CIC reset : Subsystem
  Complex Multiplier 6.0 {1..4} (4 alike) : xbsIndex_r4/Complex Multiplier 6.0   hasatlast=off  hasatuser=off  atuserwidth=1  hasbtlast=off  hasbtuser=off  btuserwidth=1  multtype=Use_Mults  optimizegoal=Resources  flowcontrol=NonBlocking  outputwidth=23  roundmode=Truncate  hasctrltlast=off  hasctrltuser=off  ctrltuserwidth=1  outtlastbehv=Null  latencyconfig=Manual  minimumlatency=6  aclken=off  aresetn=off  trim_axipin_name=on  simulation_type=hybrid_sim  simulation_model=sysgen:cmpy_v6_0  data_path_portlist={ 's_axis_a_tdata_real', 's_axis_a_tdata_imag', 's_axis_b_tdata_real', 's_axis_b_tdata_imag', 's_axis_ctrl_tdata_rounding_bit', 'm_axis_dout_tdata_real', 'm_axis_dout_tdata_imag' }  aportwidth=63  bportwidth=63  ip_name=Complex Multiplier  ip_version=6.0  dsptool_ready=true  ipcore_usecache=true  ipcore_useipmodelcache=true  ipcore_verbose=false  ipcore_latency_parameter='minimumlatency'  wrapper_available=true  port_translation_map={ 'aclken' => 'en', 'aresetn' => 'rst'}  block_type=cmpy_v6_0
  Constant : xbsIndex_r4/Constant  const=1.0  gui_display_data_type=Boolean  arith_type=Boolean  n_bits=16  bin_pt=14  preci_type=Single  exp_width=8  frac_width=24  explicit_period=off  period=1  equ=P=C  opselect=C  inp2=PCIN>>17  opr=+  inp1=P  carry=CIN  dbl_ovrd=off  block_type=constant
  Constant1 : xbsIndex_r4/Constant  const=15  gui_display_data_type=Fixed-point  arith_type=Unsigned  n_bits=4  bin_pt=0  preci_type=Single  exp_width=8  frac_width=24  explicit_period=off  period=1  equ=P=C  opselect=C  inp2=PCIN>>17  opr=+  inp1=P  carry=CIN  dbl_ovrd=off  block_type=constant
  Constant2 : xbsIndex_r4/Constant  const=1.0  gui_display_data_type=Boolean  arith_type=Boolean  n_bits=16  bin_pt=14  preci_type=Single  exp_width=8  frac_width=24  explicit_period=off  period=1  equ=P=C  opselect=C  inp2=PCIN>>17  opr=+  inp1=P  carry=CIN  dbl_ovrd=off  block_type=constant
  Constant4 : xbsIndex_r4/Constant  const=10  gui_display_data_type=Fixed-point  arith_type=Unsigned  n_bits=4  bin_pt=0  preci_type=Single  exp_width=8  frac_width=24  explicit_period=off  period=1  equ=P=C  opselect=C  inp2=PCIN>>17  opr=+  inp1=P  carry=CIN  dbl_ovrd=off  block_type=constant
  Constant6 : xbsIndex_r4/Constant  const=1.0  gui_display_data_type=Boolean  arith_type=Boolean  n_bits=16  bin_pt=14  preci_type=Single  exp_width=8  frac_width=24  explicit_period=off  period=1  equ=P=C  opselect=C  inp2=PCIN>>17  opr=+  inp1=P  carry=CIN  dbl_ovrd=off  block_type=constant
  Convert{,1..7} (8 alike) : xbsIndex_r4/Convert  gui_display_data_type=Fixed-point  arith_type="Signed  (2's comp)"  n_bits=20  bin_pt=18  float_type=Single  exp_bits=8  fraction_bits=24  quantization="Round  (unbiased: +/- Inf)"  overflow=Saturate  en=off  latency=0  pipeline=off  dbl_ovrd=off  block_type=convert
  Delay{1..5} (5 alike) : xbsIndex_r4/Delay  rst=off  infoeditControl=Selection of Reset will increase slice count due to use of real FFs and instead of SRLs  en=off  latency=6  reg_retiming=off  dbl_ovrd=off  block_type=delay
  Delay6 : xbsIndex_r4/Delay  rst=off  infoeditControl=Selection of Reset will increase slice count due to use of real FFs and instead of SRLs  en=off  latency=8  reg_retiming=off  dbl_ovrd=off  block_type=delay
  Demux{,1,3..4} (4 alike) : Demux  Outputs=2
  Demux2 : Demux  Outputs=14
  Gateway Out{1..14} (14 alike) : xbsIndex_r4/Gateway Out  inherit_from_input=off  hdl_port=off  rows=1  columns=1  UseAsDAC=off  DACChannel='1'  interface=None  automatic_assignment=on  address_offset=hex2dec('00')  intf_name=''  intf_description=''  timing_constraint=None  locs_specified=off  LOCs={}  io_standard={}  block_type=gatewayout
  Mux : Mux  Inputs=6
  Mux{1..13} (13 alike) : Mux  Inputs=2
  Mux14 : xbsIndex_r4/Mux  inputs=2  en=off  latency=0  precision=Full  arith_type=Unsigned  n_bits=16  bin_pt=14  quantization=Truncate  overflow=Wrap  dbl_ovrd=off  block_type=mux
  Negate : xbsIndex_r4/Negate  precision=User Defined  arith_type="Signed  (2's comp)"  n_bits=16  bin_pt=14  quantization=Truncate  overflow=Wrap  en=off  latency=0  dbl_ovrd=off  block_type=negate
  Negate1 : xbsIndex_r4/Negate  precision=User Defined  arith_type="Signed  (2's comp)"  n_bits=16  bin_pt=14  quantization=Truncate  overflow=Wrap  en=off  latency=0  dbl_ovrd=off  block_type=negate
  Scale{1..12} (12 alike) : xbsIndex_r4/Scale  scale_factor=-11  dbl_ovrd=off  block_type=scale
  AllComponents : Outport
  wires:
  "CIC Compiler 4.0 "/3 -> Scale1/1
  Demux/1 -> Demux1/1
  Demux1/1 -> Delay2/1, Complex Multiplier 6.0 4/2, Complex Multiplier 6.0 1/2
  Demux1/2 -> Complex Multiplier 6.0 4/3, Delay1/1, Complex Multiplier 6.0 1/3
  Demux/2 -> Demux4/1
  [SBI] -> Complex Multiplier 6.0 4/6
  [SBQ] -> Complex Multiplier 6.0 4/5
  CIC reset/2(tlast) -> CIC Compiler 4.0 2/3, CIC Compiler 4.0 8/3, CIC Compiler 4.0 10/3, CIC Compiler 4.0 11/3, CIC Compiler 4.0 9/3, CIC Compiler 4.0 7/3, CIC Compiler 4.0 6/3, CIC Compiler 4.0 5/3, CIC Compiler 4.0 4/3, CIC Compiler 4.0 3/3, CIC Compiler 4.0 1/3, "CIC Compiler 4.0 "/3
  CIC reset/1(notResetOut) -> CIC Compiler 4.0 2/1, CIC Compiler 4.0 3/4, CIC Compiler 4.0 7/4, CIC Compiler 4.0 8/4, CIC Compiler 4.0 11/4, CIC Compiler 4.0 10/4, CIC Compiler 4.0 9/4, CIC Compiler 4.0 6/4, CIC Compiler 4.0 5/4, CIC Compiler 4.0 4/4, CIC Compiler 4.0 2/4, CIC Compiler 4.0 1/4, "CIC Compiler 4.0 "/4
  In1/1 -> Demux3/1
  Demux3/2 -> Demux/1
  Delay1/1 -> CIC Compiler 4.0 1/2
  Delay2/1 -> "CIC Compiler 4.0 "/2
  CIC Compiler 4.0 1/3 -> Scale2/1
  CIC Compiler 4.0 2/3 -> Scale3/1
  Complex Multiplier 6.0 4/2 -> Convert3/1
  Complex Multiplier 6.0 4/3 -> Convert2/1
  Complex Multiplier 6.0 1/2 -> Convert1/1
  Complex Multiplier 6.0 1/3 -> Convert/1
  Constant2/1 -> Complex Multiplier 6.0 4/4, Complex Multiplier 6.0 1/4, Complex Multiplier 6.0 1/1, Complex Multiplier 6.0 4/1
  Demux4/1 -> Complex Multiplier 6.0 2/2, Complex Multiplier 6.0 3/2, Delay5/1
  Demux4/2 -> Complex Multiplier 6.0 2/3, Complex Multiplier 6.0 3/3, Delay4/1
  [SBI] -> Complex Multiplier 6.0 3/6
  [SBQ] -> Complex Multiplier 6.0 3/5
  Constant/1 -> "CIC Compiler 4.0 "/1, CIC Compiler 4.0 4/1, CIC Compiler 4.0 11/1, CIC Compiler 4.0 10/1, CIC Compiler 4.0 9/1, CIC Compiler 4.0 8/1, CIC Compiler 4.0 7/1, CIC Compiler 4.0 6/1, CIC Compiler 4.0 5/1, CIC Compiler 4.0 3/1, CIC Compiler 4.0 1/1
  Delay4/1 -> CIC Compiler 4.0 7/2
  Delay5/1 -> CIC Compiler 4.0 6/2
  Complex Multiplier 6.0 3/2 -> Convert5/1
  Complex Multiplier 6.0 3/3 -> Convert4/1
  Complex Multiplier 6.0 2/2 -> Convert6/1
  Complex Multiplier 6.0 2/3 -> Convert7/1
  Constant6/1 -> Complex Multiplier 6.0 3/4, Complex Multiplier 6.0 2/4, Complex Multiplier 6.0 2/1, Complex Multiplier 6.0 3/1
  CIC Compiler 4.0 11/3 -> Scale12/1
  CIC Compiler 4.0 3/3 -> Scale4/1
  CIC Compiler 4.0 4/3 -> Scale5/1
  CIC Compiler 4.0 5/3 -> Scale6/1
  CIC Compiler 4.0 6/3 -> Scale7/1
  CIC Compiler 4.0 7/3 -> Scale8/1
  CIC Compiler 4.0 8/3 -> Scale9/1
  CIC Compiler 4.0 9/3 -> Scale10/1
  CIC Compiler 4.0 10/3 -> Scale11/1
  Demux3/1 -> Delay3/1, [ChanIn]
  Delay3/1 -> CIC reset/2(Channel)
  Scale2/1 -> Mux1/2
  Scale1/1 -> Mux1/1
  Scale4/1 -> Mux2/2
  Scale3/1 -> Mux2/1
  Scale6/1 -> Mux3/2
  Scale5/1 -> Mux3/1
  Scale7/1 -> Mux4/1
  Scale8/1 -> Mux4/2
  Scale9/1 -> Mux5/1
  Scale10/1 -> Mux5/2
  Scale11/1 -> Mux6/1
  Scale12/1 -> Mux6/2
  Mux6/1 -> Mux/6
  Mux5/1 -> Mux/5
  Mux4/1 -> Mux/4
  Mux3/1 -> Mux/3
  Mux2/1 -> Mux/2
  Mux1/1 -> Mux/1
  Mux/1 -> Bus Creator/2
  [ChanIn] -> Delay6/1  "channel"
  CIC Compiler 4.0 6/2 -> Mux14/1, Bus Creator1/2  "valid"
  Bus Creator1/1 -> Bus Creator/1  "chanAndTvalid"
  Convert/1 -> CIC Compiler 4.0 5/2
  Convert1/1 -> CIC Compiler 4.0 4/2
  Convert2/1 -> CIC Compiler 4.0 3/2
  Convert3/1 -> CIC Compiler 4.0 2/2
  Convert4/1 -> CIC Compiler 4.0 9/2
  Convert5/1 -> CIC Compiler 4.0 8/2
  Convert7/1 -> CIC Compiler 4.0 11/2
  Convert6/1 -> CIC Compiler 4.0 10/2
  Bus Creator/1 -> AllComponents/1, Demux2/1
  Demux2/1 -> Gateway Out3/1
  Demux2/2 -> Gateway Out4/1
  Demux2/3 -> Gateway Out5/1
  Demux2/4 -> Gateway Out6/1
  Gateway Out6/1 -> Mux8/2
  Gateway Out5/1 -> Mux8/1
  Gateway Out4/1 -> Mux7/2
  Gateway Out3/1 -> Mux7/1
  Mux7/1 -> 1c demod Scope/1
  Mux8/1 -> 1c demod Scope/2
  Demux2/14 -> Gateway Out14/1
  Demux2/13 -> Gateway Out13/1
  Gateway Out13/1 -> Mux13/1
  Gateway Out14/1 -> Mux13/2
  Mux13/1 -> 1c demod Scope/7
  Demux2/12 -> Gateway Out12/1
  Demux2/11 -> Gateway Out11/1
  Gateway Out11/1 -> Mux12/1
  Gateway Out12/1 -> Mux12/2
  Mux12/1 -> 1c demod Scope/6
  Demux2/10 -> Gateway Out10/1
  Demux2/9 -> Gateway Out9/1
  Gateway Out9/1 -> Mux11/1
  Gateway Out10/1 -> Mux11/2
  Mux11/1 -> 1c demod Scope/5
  Demux2/8 -> Gateway Out8/1
  Gateway Out8/1 -> Mux10/2
  Mux10/1 -> 1c demod Scope/4
  Gateway Out7/1 -> Mux10/1
  Demux2/7 -> Gateway Out7/1
  Demux2/6 -> Gateway Out2/1
  Gateway Out2/1 -> Mux9/2
  Gateway Out1/1 -> Mux9/1
  Demux2/5 -> Gateway Out1/1
  Mux9/1 -> 1c demod Scope/3
  Constant4/1 -> CIC reset/3(N-2)
  [fpgaReset] -> CIC reset/1(resetIn)
  Delay6/1 -> Mux14/3  "channel"
  Constant1/1 -> Mux14/2
  Mux14/1 -> Bus Creator1/1  "channel"
  [SBI] -> Complex Multiplier 6.0 1/6
  Negate/1 -> Complex Multiplier 6.0 1/5
  [SBQ] -> Negate/1
  [SBI] -> Complex Multiplier 6.0 2/6
  [SBQ] -> Negate1/1
  Negate1/1 -> Complex Multiplier 6.0 2/5
